simulink model "Trial_with_intermediate_tanks"  (R2023b)
settings: Solver=ode23s  StartTime=0.0  StopTime=0.2  FixedStep=1e-6  MaxStep=1e-6  RelTol=1e-8
InitFcn:
  | param = struct();
  | 
  | param.P_H = 20e6;
  | param.P_M = 10e6;
  | param.P_L = 101325;
  | 
  | % Linear Actuator Chamber
  | param.V1_0 = 1e-3;
  | param.Acap = 0.0045;
  | 
  | % Intermediary volumes
  | param.V3_0 = 200e-6;
  | param.V4_0 = 200e-6;
  | 
  | % Fluid
  | param.beta = 1.8e9;
  | 
  | % Valve
  | param.max_Avt = 0.5*0.25*pi*(20e-3)^2;
  | param.Cd = 0.6;
  | 
  | % Valve Dynamics
  | param.wn = 50*2*pi;
  | param.zeta = 1;
  | 
  | % Hydraulic Pump/Motor
  | param.J_hyd = 3000e-7;
  | param.D = 1.61e-6;    % In cc/rev
  | 
  | % Electric Motor/Generator
  | param.J_elec = 1530e-7;
settings Model: SimulationMode=rapid-accelerator  Creator=ibrah408  LastModifiedBy=ibrah408
settings SolverCC: MaxConsecutiveZCs=10000

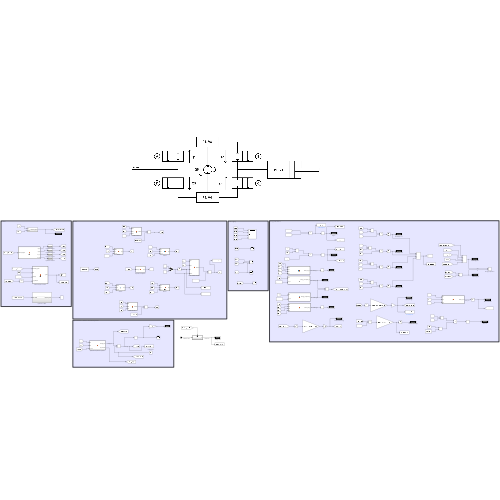
[thumbnail: Simulink's stored preview of the top-level diagram]
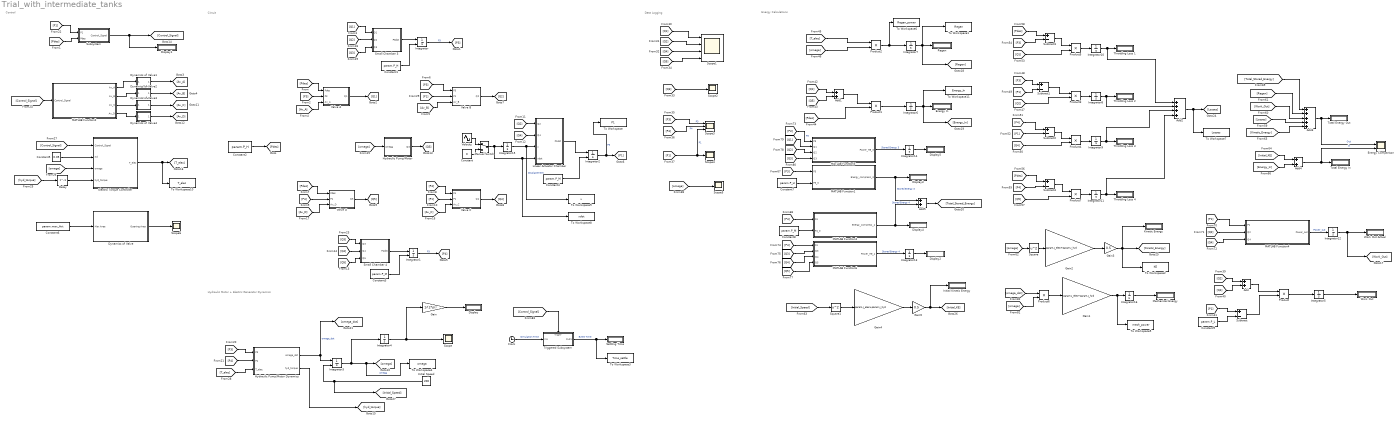
== system Trial_with_intermediate_tanks ==
  note: Energy Calculations
  note: Data Logging
  note: Hydraulic Motor + Electric Generator Dynamics
  note: Circuit
  note: Control
  Add{,1,4..5} (4 alike) : Sum
  Add2 : Sum  Inputs=++++
  Add3 : Sum  Inputs=+++++
  Clock : Clock
  Constant : Constant  Value=0
  Constant1 : Constant  Value=param.P_H
  Constant2 : Constant  Value=param.P_H
  Constant3 : Constant  Value=param.P_M
  Constant4 : Constant  Value=param.P_M
  Constant5 : Constant  Value=0.05
  Constant6 : Constant  Value=param.max_Avt
  Constant7 : Constant  Value=param.P_H
  Constant8 : Constant  Value=param.P_M
  Constant9 : Constant  Value=param.P_L
  Delay : Delay  DelayLength=1
  Display{,1..5} (6 alike) : Display
  Dynamics of Valve : Subsystem
  Dynamics of Valve1 : Subsystem
  Dynamics of Valve2 : Subsystem
  Dynamics of Valve3 : Subsystem
  Dynamics of Valve4 : Subsystem
  Electric Torque Controller : MATLAB Function  TreatAsAtomicUnit=on
  Energy Comparison : Scope  NumInputPorts=2
  Energy In : Display
  Gain : Gain  Gain=1/(2*pi)
  Gain1 : Gain  Gain=param.J_elec+param.J_hyd
  Gain2 : Gain  Gain=param.J_elec+param.J_hyd
  Gain3 : Gain  Gain=0.5
  Gain4 : Gain  Gain=param.J_elec+param.J_hyd
  Gain5 : Gain  Gain=0.5
  Hydraulic Pump/Motor : MATLAB Function  TreatAsAtomicUnit=on
  Hydraulic Pump/Motor Dynamics : MATLAB Function  TreatAsAtomicUnit=on
  Initial Kinetic Energy : Display
  Initial Speed : Constant  Value=200
  Integrator : Integrator  InitialConditionSource=external  InitialCondition=param.P_M
  Integrator1 : Integrator  InitialConditionSource=external  InitialCondition=param.P_M
  Integrator{4..16} (13 alike) : Integrator
  Integrator2 : Integrator  InitialConditionSource=external  InitialCondition=param.P_M
  Integrator3 : Integrator  InitialConditionSource=external
  Kinetic Energy : Display
  Linear Actuator Chamber : MATLAB Function  TreatAsAtomicUnit=on
  MATLAB Function1 : MATLAB Function  TreatAsAtomicUnit=on
  MATLAB Function2 : MATLAB Function  TreatAsAtomicUnit=on
  MATLAB Function3 : MATLAB Function  TreatAsAtomicUnit=on
  MATLAB Function4 : MATLAB Function  TreatAsAtomicUnit=on
  MATLAB Function5 : MATLAB Function  TreatAsAtomicUnit=on
  MATLAB Function6 : MATLAB Function  TreatAsAtomicUnit=on
  Manual Switch : ManualSwitch
  Mechanical Energy : Display
  Product{,1..7} (8 alike) : Product
  Regen : Display
  Scope{,2,4..6} (5 alike) : Scope
  Scope1 : Scope  NumInputPorts=4
  Scope3 : Scope  NumInputPorts=3
  Settling Time : Display
  Small Chamber 3 : MATLAB Function  TreatAsAtomicUnit=on
  Small Chamber 4 : MATLAB Function  TreatAsAtomicUnit=on
  Square : Math  Operator=square
  Square1 : Math  Operator=square
  Subsystem : Subsystem
  Subtract{,1..4} (5 alike) : Sum  Inputs=+-
  Throttling Loss {1..4} (4 alike) : Display
  To Workspace : ToWorkspace  VariableName=P1  SaveFormat=Timeseries  SampleTime=-1
  To Workspace1 : ToWorkspace  VariableName=Regen  SaveFormat=Timeseries  SampleTime=-1
  To Workspace10 : ToWorkspace  VariableName=T_elec  SaveFormat=Timeseries  SampleTime=-1
  To Workspace11 : ToWorkspace  VariableName=Energy_In  SaveFormat=Timeseries  SampleTime=-1
  To Workspace2 : ToWorkspace  VariableName=KE  SaveFormat=Timeseries  SampleTime=-1
  To Workspace3 : ToWorkspace  VariableName=Time_settle  SaveFormat=Timeseries  SampleTime=-1
  To Workspace4 : ToWorkspace  VariableName=omega  SaveFormat=Timeseries  SampleTime=-1
  To Workspace5 : ToWorkspace  VariableName=mech_power  SaveFormat=Timeseries  SampleTime=-1
  To Workspace6 : ToWorkspace  VariableName=Regen_power  SaveFormat=Timeseries  SampleTime=-1
  To Workspace7 : ToWorkspace  VariableName=Losses  SaveFormat=Timeseries  SampleTime=-1
  To Workspace8 : ToWorkspace  VariableName=xdot  SaveFormat=Timeseries  SampleTime=-1
  To Workspace9 : ToWorkspace  VariableName=x  SaveFormat=Timeseries  SampleTime=-1
  Total Energy In : Display
  Total Energy Out : Display
  Triggered Subsystem : Subsystem  TreatAsAtomicUnit=on
  Valve A : MATLAB Function  TreatAsAtomicUnit=on
  Valve B : MATLAB Function  TreatAsAtomicUnit=on
  Valve C : MATLAB Function  TreatAsAtomicUnit=on
  Valve D : MATLAB Function  TreatAsAtomicUnit=on
  Velocity : Sin  Amplitude=1e-2  Frequency=(2*pi)/0.2  Phase=pi/2  SampleTime=0
  Work Out : Display
  Work Out Actual : Display
  wires:
  [Pdes] -> Valve A/1(Pdes)
  Small Chamber 3/1(P3dot) -> Integrator/1
  Constant1/1 -> Integrator/2
  Constant2/1 -> [Pdes]
  [Pdes] -> Subsystem/2(Pdes)
  Integrator/1 -> [P3]  "P3"
  [P3] -> Valve A/2(P3)
  Valve A/1(Q1) -> [Q1]
  [Q1] -> Small Chamber 3/1(Q1)
  [Av_A] -> Valve A/3(Av_A)
  [Av_B] -> Valve B/3(Av_B)
  [P3] -> Valve B/1(P3)
  [Pdes] -> Valve D/1(Pdes)
  Small Chamber 4/1(P4dot) -> Integrator1/1
  Constant3/1 -> Integrator1/2
  Integrator1/1 -> [P4]  "P3"
  [P4] -> Valve C/1(P4)
  [P4] -> Valve D/2(P4)
  Linear Actuator Chamber/1(P1dot) -> Integrator2/1
  Constant4/1 -> Integrator2/2
  Integrator2/1 -> To Workspace/1, [P1]  "P3"
  [P1] -> Valve C/2(P1)
  Valve B/1(Q2) -> [Q2]
  [Q2] -> Linear Actuator Chamber/1(Q2)
  Valve C/1(Q4) -> [Q4]
  [Q4] -> Linear Actuator Chamber/2(Q4)
  Valve D/1(Q5) -> [Q5]
  [Q5] -> Small Chamber 4/3(Q5)
  [Q4] -> Small Chamber 4/2(Q4)
  Hydraulic Pump/Motor Dynamics/1(omega_dot) -> [omega_dot], Integrator3/1  "omega_dot"
  Initial Speed/1 -> [Initial_Speed], Integrator3/2
  Integrator3/1 -> Integrator4/1, To Workspace4/1, [omega]  "omega"
  [omega] -> Hydraulic Pump/Motor/1(omega)
  [Av_C] -> Valve C/3(Av_C)
  [Av_D] -> Valve D/3(Av_D)
  [Q2] -> Small Chamber 3/2(Q2)
  Hydraulic Pump/Motor/1(Q3) -> [Q3]
  [Q3] -> Small Chamber 3/3(Q3)
  [P3] -> Hydraulic Pump/Motor Dynamics/1(P3)
  [P4] -> Hydraulic Pump/Motor Dynamics/2(P4)
  [P1] -> Subsystem/1(P1)
  [Q3] -> Small Chamber 4/1(Q3)
  Subsystem/1(Control_Signal) -> [Control_Signal], Display1/1
  [Control_Signal] -> MATLAB Function2/1(Control_Signal)
  Integrator4/1 -> Gain/1, Scope/1
  Gain/1 -> Display/1
  Hydraulic Pump/Motor Dynamics/2(hyd_torque) -> [hyd_torque]
  [hyd_torque] -> Delay/1
  Delay/1 -> Electric Torque Controller/4(hyd_torque)
  [omega] -> Electric Torque Controller/3(omega)
  Constant5/1 -> Electric Torque Controller/2(Kd)
  [Control_Signal] -> Electric Torque Controller/1(Control_Signal)
  Electric Torque Controller/1(T_elec) -> To Workspace10/1, [T_elec]
  [T_elec] -> Hydraulic Pump/Motor Dynamics/3(T_elec)
  [P1] -> Valve B/2(P1)
  [Q1] -> Scope1/1
  [Q2] -> Scope1/2
  [Q4] -> Scope1/3
  [Q5] -> Scope1/4
  [Q3] -> Scope2/1
  [P3] -> Scope3/1  "P3"
  [P4] -> Scope3/2  "P4"
  [P1] -> Scope3/3, Scope4/1  "P1"
  [omega] -> Scope5/1
  [Q4] -> Add/2
  [Q2] -> Add/1
  Add/1 -> Product/1
  Product/1 -> Integrator5/1
  Integrator5/1 -> Work Out/1
  [Q1] -> Add1/1
  [Q5] -> Add1/2
  Add1/1 -> Product1/1
  [Pdes] -> Product1/2
  Product1/1 -> Integrator6/1
  Integrator6/1 -> To Workspace11/1, [Energy_In], Energy In/1
  [T_elec] -> Product2/1
  [omega] -> Product2/2
  Product2/1 -> To Workspace6/1, Integrator7/1
  Integrator7/1 -> To Workspace1/1, [Regen], Regen/1
  Constant6/1 -> Dynamics of Valve/1(Max Area)
  Dynamics of Valve/1(Opening Area) -> Scope6/1
  MATLAB Function2/1(Av_A) -> Dynamics of Valve1/1(Max Area)
  Dynamics of Valve1/1(Opening Area) -> [Av_A]
  MATLAB Function2/2(Av_B) -> Dynamics of Valve2/1(Max Area)
  Dynamics of Valve2/1(Opening Area) -> [Av_B]
  MATLAB Function2/3(Av_C) -> Dynamics of Valve3/1(Max Area)
  Dynamics of Valve3/1(Opening Area) -> [Av_C]
  MATLAB Function2/4(Av_D) -> Dynamics of Valve4/1(Max Area)
  Dynamics of Valve4/1(Opening Area) -> [Av_D]
  Product4/1 -> Integrator9/1
  [Q2] -> Product3/2
  [P4] -> Subtract2/1
  Integrator11/1 -> Add2/4, Throttling Loss 4/1
  [P4] -> Subtract4/2
  [Pdes] -> Subtract4/1
  [P1] -> Subtract2/2
  Product7/1 -> Integrator11/1
  Integrator9/1 -> Add2/3, Throttling Loss 3/1
  Subtract3/1 -> Product5/1
  Product3/1 -> Integrator8/1
  [Pdes] -> Subtract3/1
  Add2/1 -> To Workspace7/1, [Losses]
  Subtract1/1 -> Product3/1
  Product5/1 -> Integrator10/1
  [P3] -> Subtract1/1
  Integrator8/1 -> Add2/2, Throttling Loss 2/1
  [P1] -> Subtract1/2
  [Q5] -> Product7/2
  Integrator10/1 -> Add2/1, Throttling Loss 1/1
  [P3] -> Subtract3/2
  Subtract4/1 -> Product7/1
  [Q4] -> Product4/2
  Subtract2/1 -> Product4/1
  [Q1] -> Product5/2
  [Regen] -> Add3/2
  [Work_Out] -> Add3/3
  [Losses] -> Add3/4
  Gain3/1 -> To Workspace2/1, [Kinetic_Energy], Kinetic Energy/1
  [omega] -> Square/1
  Square/1 -> Gain2/1
  Gain2/1 -> Gain3/1
  [Initial_Speed] -> Square1/1
  Gain4/1 -> Gain5/1
  Square1/1 -> Gain4/1
  Gain5/1 -> Initial Kinetic Energy/1, [Initial_KE]
  [Kinetic_Energy] -> Add3/5
  [Initial_KE] -> Add4/1
  [Energy_In] -> Add4/2
  Add4/1 -> Energy Comparison/2, Total Energy In/1  "In"
  Add3/1 -> Energy Comparison/1, Total Energy Out/1  "Out"
  Constant7/1 -> MATLAB Function1/2(P3_0)
  [P3] -> MATLAB Function1/1(P3)
  [P4] -> MATLAB Function3/1(P4)
  Constant8/1 -> MATLAB Function3/2(P4_0)
  MATLAB Function1/1(Energy_compress_3) -> Display3/1, Add5/1  "Stored Energy 3"
  MATLAB Function3/1(Energy_compress_4) -> Display4/1, Add5/2  "Stored Energy 4"
  Add5/1 -> [Total_Stored_Energy]
  [Total_Stored_Energy] -> Add3/1
  [P1] -> MATLAB Function4/1(P1)
  MATLAB Function4/1(Power_out) -> Integrator12/1  "Power_out"
  [Q4] -> MATLAB Function4/3(Q4)
  [Q2] -> MATLAB Function4/2(Q2)
  Integrator12/1 -> [Work_Out], Work Out Actual/1
  [P1] -> Subtract/1
  Constant9/1 -> Subtract/2
  Subtract/1 -> Product/2
  [P4] -> MATLAB Function6/1(P4)
  [Q3] -> MATLAB Function6/2(Q3)
  [Q4] -> MATLAB Function6/3(Q4)
  [Q5] -> MATLAB Function6/4(Q5)
  MATLAB Function6/1(Power_HE_4) -> Integrator13/1  "Stored Energy 4"
  Integrator13/1 -> Display2/1
  Integrator14/1 -> Display5/1
  MATLAB Function5/1(Power_HE_3) -> Integrator14/1  "Stored Energy 3"
  [Q1] -> MATLAB Function5/2(Q1)
  [P3] -> MATLAB Function5/1(P3)  "P3"
  [Q2] -> MATLAB Function5/3(Q2)
  [Q3] -> MATLAB Function5/4(Q3)
  Integrator15/1 -> To Workspace9/1, Linear Actuator Chamber/3(x)  "Displacement"
  Velocity/1 -> Manual Switch/1
  Manual Switch/1 -> To Workspace8/1, Linear Actuator Chamber/4(xdot), Integrator15/1
  Constant/1 -> Manual Switch/2
  Product6/1 -> Gain1/1
  [omega] -> Product6/2
  Integrator16/1 -> Mechanical Energy/1
  [omega_dot] -> Product6/1
  Gain1/1 -> To Workspace5/1, Integrator16/1
  [Control_Signal] -> Triggered Subsystem/Trigger
  Clock/1 -> Triggered Subsystem/1(In1)  "Simulation Time"
  Triggered Subsystem/1(Out1) -> To Workspace3/1, Settling Time/1  "Event Time"

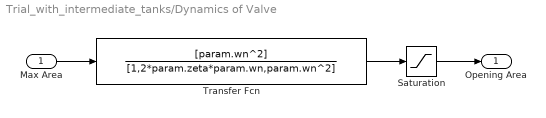
== system Trial_with_intermediate_tanks/Dynamics of Valve ==
  Max Area : Inport
  Saturation : Saturate  UpperLimit=param.max_Avt  LowerLimit=0
  Transfer Fcn : TransferFcn  Numerator=[param.wn^2]  Denominator=[1,2*param.zeta*param.wn,param.wn^2]
  Opening Area : Outport
  wires:
  Transfer Fcn/1 -> Saturation/1
  Saturation/1 -> Opening Area/1
  Max Area/1 -> Transfer Fcn/1

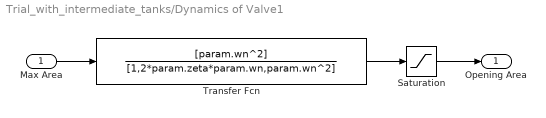
== system Trial_with_intermediate_tanks/Dynamics of Valve1 ==
  Max Area : Inport
  Saturation : Saturate  UpperLimit=param.max_Avt  LowerLimit=0
  Transfer Fcn : TransferFcn  Numerator=[param.wn^2]  Denominator=[1,2*param.zeta*param.wn,param.wn^2]
  Opening Area : Outport
  wires:
  Max Area/1 -> Transfer Fcn/1
  Saturation/1 -> Opening Area/1
  Transfer Fcn/1 -> Saturation/1

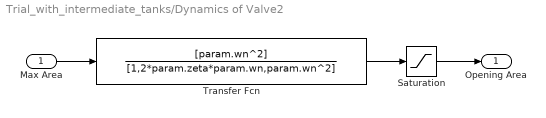
== system Trial_with_intermediate_tanks/Dynamics of Valve2 ==
  Max Area : Inport
  Saturation : Saturate  UpperLimit=param.max_Avt  LowerLimit=0
  Transfer Fcn : TransferFcn  Numerator=[param.wn^2]  Denominator=[1,2*param.zeta*param.wn,param.wn^2]
  Opening Area : Outport
  wires:
  Transfer Fcn/1 -> Saturation/1
  Saturation/1 -> Opening Area/1
  Max Area/1 -> Transfer Fcn/1

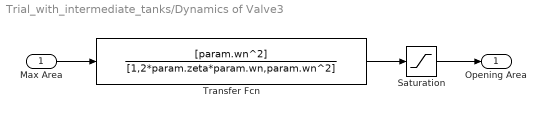
== system Trial_with_intermediate_tanks/Dynamics of Valve3 ==
  Max Area : Inport
  Saturation : Saturate  UpperLimit=param.max_Avt  LowerLimit=0
  Transfer Fcn : TransferFcn  Numerator=[param.wn^2]  Denominator=[1,2*param.zeta*param.wn,param.wn^2]
  Opening Area : Outport
  wires:
  Max Area/1 -> Transfer Fcn/1
  Saturation/1 -> Opening Area/1
  Transfer Fcn/1 -> Saturation/1

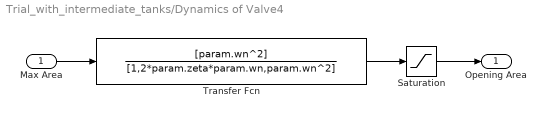
== system Trial_with_intermediate_tanks/Dynamics of Valve4 ==
  Max Area : Inport
  Saturation : Saturate  UpperLimit=param.max_Avt  LowerLimit=0
  Transfer Fcn : TransferFcn  Numerator=[param.wn^2]  Denominator=[1,2*param.zeta*param.wn,param.wn^2]
  Opening Area : Outport
  wires:
  Transfer Fcn/1 -> Saturation/1
  Saturation/1 -> Opening Area/1
  Max Area/1 -> Transfer Fcn/1

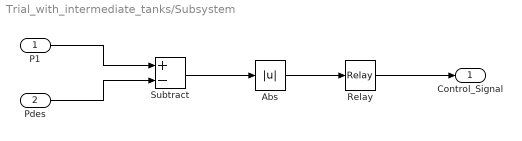
== system Trial_with_intermediate_tanks/Subsystem ==
  P1 : Inport
  Pdes : Inport  Port=2
  Abs : Abs  SaturateOnIntegerOverflow=off
  Relay : Relay  OnSwitchValue=1e6  OffSwitchValue=1e4  OnOutputValue=0  OffOutputValue=1
  Subtract : Sum  Inputs=+-
  Control_Signal : Outport
  wires:
  P1/1 -> Subtract/1
  Pdes/1 -> Subtract/2
  Subtract/1 -> Abs/1
  Abs/1 -> Relay/1
  Relay/1 -> Control_Signal/1

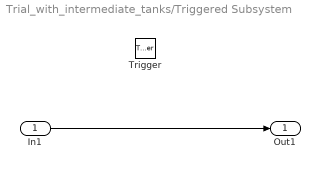
== system Trial_with_intermediate_tanks/Triggered Subsystem ==
  In1 : Inport
  Trigger : TriggerPort  VariantControl=(inherit)
  Out1 : Outport
  wires:
  In1/1 -> Out1/1

== matlab function Trial_with_intermediate_tanks/Hydraulic Pump//Motor Dynamics ==
  data: P3 input; omega_dot output; P4 input; T_elec input; param parameter; hyd_torque output
function [omega_dot, hyd_torque] = fcn(P3,P4,T_elec,param)

hyd_torque = (param.D/(2*pi))*(P3-P4);
omega_dot = (1/(param.J_elec+param.J_hyd))*(hyd_torque-T_elec);

== matlab function Trial_with_intermediate_tanks/Electric Torque Controller ==
  data: Control_Signal input; Kd input; omega input; hyd_torque input; T_elec output
function T_elec  = fcn(Control_Signal, Kd, omega, hyd_torque)

if Control_Signal == 1 

    if omega < 200
        T_elec = hyd_torque;
    else
        T_elec = 5;
    end

else

    if omega >= 300
        T_elec = hyd_torque;
    else
        T_elec = -5;
    end

end

== matlab function Trial_with_intermediate_tanks/MATLAB Function3 ==
  data: P4 input; P4_0 input; Energy_compress_4 output; param parameter
function Energy_compress_4  = fcn(P4, P4_0, param)

%% Normal
Pg = P4 - param.P_L;
P0 = P4_0 - param.P_L;

Wv = param.beta*(exp(Pg/param.beta)-(1+Pg/param.beta));
W0 = param.beta*(exp(P0/param.beta)-(1+P0/param.beta));

Energy_compress_4 = param.V4_0*(Wv-W0);

== matlab function Trial_with_intermediate_tanks/MATLAB Function1 ==
  data: P3 input; P3_0 input; Energy_compress_3 output; param parameter
function Energy_compress_3  = fcn(P3, P3_0, param)

%% Normal
Pg = P3 - param.P_L;
P0 = P3_0 - param.P_L;

Wv = param.beta*(exp(Pg/param.beta)-(1+Pg/param.beta));
W0 = param.beta*(exp(P0/param.beta)-(1+P0/param.beta));

Energy_compress_3 = param.V3_0*(Wv-W0);

== matlab function Trial_with_intermediate_tanks/MATLAB Function4 ==
  data: P1 input; Power_out output; param parameter; Q2 input; Q4 input
function Power_out  = fcn(P1, param, Q2, Q4)

%% Normal
Pg = P1-param.P_L;
Wv = param.beta*(exp(Pg/param.beta)-(1+Pg/param.beta));

Power_out = (Q2+Q4)*(Wv+Pg);

== matlab function Trial_with_intermediate_tanks/MATLAB Function5 ==
  data: P3 input; param parameter; Q1 input; Q2 input; Q3 input; Power_HE_3 output
function Power_HE_3  = fcn(P3, param, Q1, Q2, Q3)

%% Hydraulic Effort
Pg = P3 - param.P_L;

phi_v = param.beta*(exp(Pg/param.beta)-1);

Power_HE_3 = (Q1-Q2-Q3)*(phi_v);

== matlab function Trial_with_intermediate_tanks/Small Chamber 3 ==
  data: P3dot output; Q1 input; Q2 input; Q3 input; param parameter
function P3dot = fcn(Q1, Q2, Q3, param)

P3dot = (param.beta/(param.V3_0))*(Q1-Q2-Q3);

== matlab function Trial_with_intermediate_tanks/MATLAB Function6 ==
  data: P4 input; param parameter; Q3 input; Power_HE_4 output; Q4 input; Q5 input
function Power_HE_4  = fcn(P4, param, Q3, Q4, Q5)

%% Hydraulic Effort
Pg = P4 - param.P_L;

phi_v = param.beta*(exp(Pg/param.beta)-1);

Power_HE_4 = (Q3+Q5-Q4)*(phi_v);

== matlab function Trial_with_intermediate_tanks/Valve A ==
  data: Pdes input; Q1 output; P3 input; Av_A input; param parameter
function Q1 = fcn(Pdes, P3, Av_A, param)

delP = Pdes - P3;
Q1 = param.Cd*Av_A*sqrt(abs(delP))*sign(delP);

== matlab function Trial_with_intermediate_tanks/MATLAB Function2 ==
  data: Control_Signal input; Av_A output; param parameter; Av_B output; Av_C output; Av_D output
function [Av_A, Av_B, Av_C, Av_D] = fcn(Control_Signal, param)

if Control_Signal==1
    
    % Phase 2
    Av_A = param.max_Avt;
    Av_B = param.max_Avt;
    Av_C = 0;
    Av_D = param.max_Avt;

else

    % Phase 1
    Av_A = param.max_Avt;
    Av_B = 0;
    Av_C = param.max_Avt;
    Av_D = 0;

end

== matlab function Trial_with_intermediate_tanks/Valve B ==
  data: Q2 output; P3 input; P1 input; Av_B input; param parameter
function Q2 = fcn(P3, P1, Av_B, param)

delP = P3 - P1;
Q2 = param.Cd*Av_B*sqrt(abs(delP))*sign(delP);

== matlab function Trial_with_intermediate_tanks/Valve D ==
  data: Pdes input; Q5 output; P4 input; Av_D input; param parameter
function Q5 = fcn(Pdes, P4, Av_D, param)

delP = Pdes - P4;
Q5 = param.Cd*Av_D*sqrt(abs(delP))*sign(delP);

== matlab function Trial_with_intermediate_tanks/Valve C ==
  data: Q4 output; P4 input; P1 input; Av_C input; param parameter
function Q4 = fcn(P4, P1, Av_C, param)

delP = P4 - P1;
Q4 = param.Cd*Av_C*sqrt(abs(delP))*sign(delP);

== matlab function Trial_with_intermediate_tanks/Small Chamber 4 ==
  data: Q3 input; P4dot output; Q4 input; Q5 input; param parameter
function P4dot = fcn(Q3, Q4, Q5, param)

P4dot = (param.beta/(param.V4_0))*(Q5+Q3-Q4);

== matlab function Trial_with_intermediate_tanks/Linear Actuator Chamber ==
  data: Q2 input; P1dot output; Q4 input; x input; xdot input; param parameter
function P1dot = fcn(Q2,Q4,x, xdot, param)

P1dot = (param.beta/(param.V1_0+param.Acap*x))*(Q2+Q4-param.Acap*xdot);

== matlab function Trial_with_intermediate_tanks/Hydraulic Pump//Motor ==
  data: omega input; Q3 output; param parameter
function Q3 = fcn(omega, param)

Q3 = (param.D/(2*pi))*omega;
